simulink model "sample04_motor_coast_encoder"  (R2023a)
settings: Solver=ode1  StartTime=0.0  StopTime=inf  FixedStep=0.005  RelTol=1e-3  EnableMultiTasking=on
libraries: drv8833lib x1, arduinosensorlib x1
settings Model: ExtModeTrigDuration=2  Creator=kawata  LastModifiedBy=kawata
settings DataIOCC: ReturnWorkspaceOutputs=off
settings OptimizationCC: EnhancedBackFolding=on  PassReuseOutputArgsAs=Individual arguments  ZeroExternalMemoryAtStartup=off  ZeroInternalMemoryAtStartup=off  MaxStackSize=64  OptimizeBlockOrder=speed  DifferentSizesBufferReuse=on  OptimizationCustomize=off  EfficientTunableParamExpr=on
settings DebuggingCC: ParameterTunabilityLossMsg=error
settings HardwareCC: ProdBitPerInt=16  ProdBitPerPointer=16  ProdBitPerSizeT=16  ProdBitPerPtrDiffT=16  ProdLargestAtomicFloat=None  ProdWordSize=8  ProdHWDeviceType=Atmel->AVR  UseEmbeddedCoderFeatures=off  UseSimulinkCoderFeatures=off
settings SFSimCC: MATLABDynamicMemAlloc=off
settings RTWCC: Description=Embedded Coder  SystemTargetFile=ert.tlc  HardwareBoard=Arduino Uno  TemplateMakefile=ert_default_tmf  Toolchain=Arduino AVR  BuildConfiguration=Faster Runs
settings CodeAppCC: ForceParamTrailComments=on  IgnoreCustomStorageClasses=off  OperatorAnnotations=on  SimulinkDataObjDesc=on  SFDataObjDesc=on  InsertBlockDesc=on
settings ERTTargetCC: SupportContinuousTime=on  SupportNonInlinedSFcns=on  SupportVariableSizeSignals=on  ExtModeTransport=3  ExtModeStaticAlloc=on  ExtModeAutomaticAllocSize=off  ExtModeStaticAllocSize=250  ExtModeMexFile=ext_xcp  ExtModeIntrfLevel=Level2 - Open

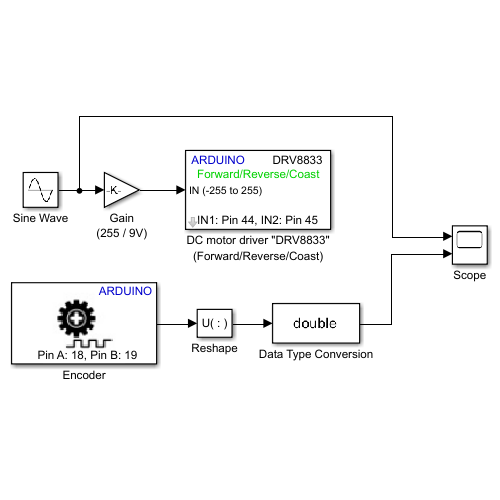
[thumbnail: Simulink's stored preview of the top-level diagram]
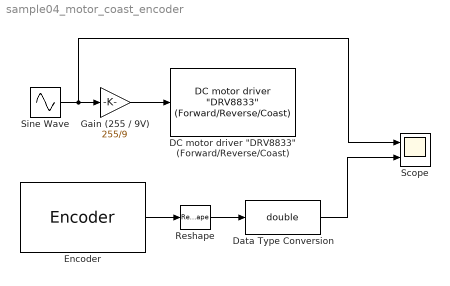
== system sample04_motor_coast_encoder ==
  "DC motor driver \"DRV8833\" (Forward/Reverse/Coast)" : drv8833lib/DC motor driver "DRV8833" (Forward//Reverse//Coast)  IN1pin=44  IN2pin=45
  Data Type Conversion : DataTypeConversion  OutDataTypeStr=double  SaturateOnIntegerOverflow=off  RndMeth=Floor
  Encoder : arduinosensorlib/Encoder  InputA=18  InputB=19  Mode=No reset  SampleTime=-1
  Gain (255 / 9V) : Gain  Gain=255/9
  Reshape : Reshape
  Scope : Scope  NumInputPorts=2
  Sine Wave : Sin  Amplitude=4  Frequency=pi/4  SampleTime=0
  wires:
  Sine Wave/1 -> Scope/1, Gain (255 / 9V)/1
  Gain (255 / 9V)/1 -> "DC motor driver \"DRV8833\" (Forward/Reverse/Coast)"/1
  Reshape/1 -> Data Type Conversion/1
  Encoder/1 -> Reshape/1
  Data Type Conversion/1 -> Scope/2
